simulink model "boost_converter_pcc"  (Simulink 7.3)
settings: Solver=ode45  StartTime=0.0  StopTime=0.1  RelTol=1e-3
InitFcn:
  | %Processor selection for I/O assignment
  | %The chosen Target in the Coder Options window must match the selected MCU.
  | %Set the variable 'type_evm' to the following strings to choose a specific target:
  | 
  |   type_evm = 'TI28379LP';  % TI28379D Delfino Launchpad
  | % type_evm = 'TI280049C';  % TI280049C Piccolo Launchpad
  | % type_evm = 'TI28379CC';  % TI28379D Delfino Controlcard
  | % type_evm = 'TI28388D';   % TI28388D Controlcard
  | 
  | 
  | % Configure I/O based on processor
  | switch (type_evm)
  | 
  | 		case 'TI28379LP'
  | 		SysClkMHz = 190;
  | 	% Configuration for TI28379D Launchpad
  | 	% on the controller side
  | 		ADC_DSP_Io = 4;
  | 		ADC_DSP_Vdc = 5;
  | 		PWM_DSP_PWM = 1;
  | 		DO_DSP_LED = 34;
  | 		DI_DSP_En = 124;
  | 		PWR_DSP_Power = 66;
  | 		SCI_DSP = [43, 42];
  | 
  | 		case 'TI280049C'
  | 		SysClkMHz = 100;
  | 	% Configuration for TI280049C Launchpad
  | 	% on the controller side
  | 		ADC_DSP_Io = 3;
  | 		ADC_DSP_Vdc = 6;
  | 		PWM_DSP_PWM = 6;
  | 		DO_DSP_LED = 34;
  | 		DI_DSP_En = 58;
  | 		PWR_DSP_Power = 56;
  | 		SCI_DSP = [28, 29];
  | 
  | 		case 'TI28379CC'
  | 		SysClkMHz = 190;
  | 	% Configuration for TI28379D Controlcard
  | 	% on the controller side
  | 	   ADC_DSP_Io = 2;
  | 		ADC_DSP_Vdc = 3;
  | 		PWM_DSP_PWM = 1;
  | 		DO_DSP_LED = 34;
  | 		DI_DSP_En = 40;
  | 		PWR_DSP_Power = 39;
  | 		SCI_DSP = [28, 29];
  | 
  | 		case 'TI28388D'
  | 		SysClkMHz = 190;
  | 	% Configuration for TI28388D Controlcard
  | 	% on the controller side
  | 	   ADC_DSP_Io = 2;
  | 		ADC_DSP_Vdc = 3;
  | 		PWM_DSP_PWM = 1;
  | 		DO_DSP_LED = 34;
  | 		DI_DSP_En = 40;
  | 		PWR_DSP_Power = 39;
  | 		SCI_DSP = [28, 29];
  | 
  | otherwise
  | 	error('Unknown evaluation module selection, please choose either ''TI28379LP'', ''TI280049C'', ''TI28379CC'' or ''TI28388D''.')
  | end
  | 
  | 
  | %Switching frequency
  | fsw = 100e3;            % in Hz
  | Ts = 1/fsw;               % in seconds
  | Ts_ctrl = Ts;
  | 
  | 
  | %Plant parameters
  | Vin = 20;                   % input voltage in V
  | Vout = 50;                 % output voltage in V
  | M = (Vout-Vin)/Vout;   % duty cycle
  | 
  | Cout = 1.5e-5;            % output capacitance in F
  | Rc = 10e-3;                % ESR of the output capacitance in Ohms
  | Rload= 20;                 % load resistance in Ohms
  | Rshunt = 0.10;           % shunt resistance in Ohms
  | 
  | %critical value of inductance
  | Lcrit = 0.5*Rload*M*(1-M)^2*Ts;
  | L = 1.5*Lcrit;               % inductance in H
  | 
  | %Ramp for peak current controller
  | ramp = (Vout-Vin)/L;
  | 
  | %Current controller Ipk calculation in CCM
  | D = M;
  | Ipk = ((Vout/Rload)/(1-D)) + 0.5*((Vout*D*(1-D)*Ts)/L);
  | 
  | SysClkHz = SysClkMHz*1e6;
  | DACq = 3.3/65536;
  | Ipk_offset = ceil(ramp*(Rshunt/DACq)*(1/SysClkHz))*(D*Ts)*(SysClkHz)*(DACq/Rshunt);
  | 
  | %Initial conditions
  | Vo_init = Vout;
  | IL_init = ((Vout/Rload)/(1-D));
  | 
  | %Designing the voltage controller using K-factor method
  | fc=1000;                       % crossover frequency in Hz
  | wc=2*pi*fc;                  % crossover frequency in rad
  | PM =60;                        % desired phase margin in degrees
  | 
  | 
  | %Analytical calculation of the phase of the plant
  | s= wc*1i;
  | %Plant transfer function
  | Gp = Rload*(1-D)*(1 - s*L/(Rload*(1-D)^2))*(1+s*Rc*Cout)/(2+s*Rload*Cout);
  | ph_sys = angle(Gp)*(180/pi);       % phase of the plant
  | 
  | 
  | %Calculate the phase boost required
  | phboost = PM - ph_sys - 90;
  | 
  | %Since the required phase boost is < 90 deg, a Type 2 controller is used
  | %Gc = Kc/s*((1+s/wz)/(1+s/wp))
  | %Calculating the poles and zeroes
  | k = tan((phboost/2+45)*pi/180);
  | wz = wc/k;
  | wp = k*wc;
  | 
  | %Analytical calculation of the gain of the controller
  | Gc = 1/s*((1+s/wz)/(1+s/wp)) ;
  | Kc=1/abs(Gc*Gp);              % gain of the controller
  | 
  | %Clear complex numbers to eliminate warning messages
  | clear('s','Gc','Gp');
undefined symbols (not defined in the file): plecs
settings Model: Creator=kris  LastModifiedBy=manaswini  ExtModeTrigMode=oneshot  ExtModeArmWhenConnect=off  ExtModeAutoUpdateStatusClock=off
settings DataIOCC: LimitDataPoints=off  ReturnWorkspaceOutputs=off  SignalLoggingName=sigsOut  Refine=10
settings OptimizationCC: BooleanDataType=off  ExpressionDepthLimit=128  InitFltsAndDblsToZero=on
settings DebuggingCC: SaveWithParameterizedLinksMsg=none  SignalResolutionControl=TryResolveAllWithWarning  SolverPrmCheckMsg=none  MultiTaskDSMMsg=warning  MultiTaskCondExecSysMsg=none  FcnCallInpInsideContextMsg=Enable All  StrictBusMsg=ErrorLevel1
settings HardwareCC: TargetHWDeviceType=32-bit Generic  TargetUnknown=on  ProdEqTarget=off
settings RTWCC: IncludeERTFirstTime=on
settings CodeAppCC: CustomSymbolStrType=$N$R$M_T
settings GRTTargetCC: TargetFcnLib=ansi_tfl_tmw.mat  TargetFunctionLibrary=C89/C90 (ANSI)  ModelReferenceCompliant=off

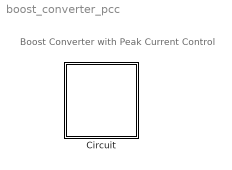
== system boost_converter_pcc ==
  note: Boost Converter with Peak Current Control
  Circuit : Subsystem  LoadFcn=plecs('sl', 200);  InitFcn=plecs('sl', 214);  StartFcn=plecs('sl', 208);  StopFcn=plecs('sl', 209);  ClipboardFcn=plecs('sl', 212, 24);  mask(PlecsCircuit){PLECSData=<binary blob, 13696 chars, not shown>}
      mask prompts: PLECSData "PLECS Data (Do not delete or modify!)"
      mask help: Drag this block into a Simulink model to create a new electrical circuit.
      mask init:
      | % PLACE CUSTOM INITIALIZATIONS ABOVE
      | % DO NOT REMOVE
      | plecs('sl', 215);
      | % DO NOT REMOVE
      settings: CopyFcn=plecs('sl', 203);  DeleteFcn=plecs('sl', 205);  UndoDeleteFcn=plecs('sl', 206);  PreSaveFcn=plecs('sl', 211);  PostSaveFcn=plecs('sl', 201);  NameChangeFcn=plecs('sl', 210);  DestroyFcn=plecs('sl', 207);  PreCopyFcn=plecs('sl', 216);  OpenFcn=plecs('sl', 202);  ErrorFcn=plerrorfcn
      mask Display: disp('PLECS\nCircuit')

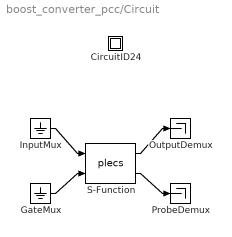
== system boost_converter_pcc/Circuit ==
  " CircuitID24 " : Subsystem
  " GateMux " : Ground
  " InputMux " : Ground
  " OutputDemux " : Terminator
  " ProbeDemux " : Terminator
  " S-Function " : S-Function  FunctionName=plecs  EnableBusSupport=off
  wires:
  " InputMux "/1 -> " S-Function "/1
  " GateMux "/1 -> " S-Function "/2
  " S-Function "/1 -> " OutputDemux "/1
  " S-Function "/2 -> " ProbeDemux "/1

== system boost_converter_pcc/Circuit/ CircuitID24  ==
